simulink model "DCDC_SEPIC_TopLevelModel_Dashboard"  (R2023b)
settings: Solver=daessc  StartTime=0.0  StopTime=10  FixedStep=ts500us  MaxStep=1  RelTol=1e-3
undefined symbols (not defined in the file): NrLEDStrips, operatingMode, ts1ms, ts500us
libraries: SEPIC_utilities x6, simulink x1
settings Model: Creator=vlenzi  LastModifiedBy=vlenzi
settings SolverCC: AlgebraicLoopSolver=TrustRegion  DecoupledContinuousIntegration=on
settings DataIOCC: SaveFormat=StructureWithTime  SaveOutput=off  SaveTime=off  SignalLoggingName=logsOut
settings OptimizationCC: DefaultParameterBehavior=Inlined  UseDivisionForNetSlopeComputation=UseDivisionForReciprocalsOfIntegersOnly  ReuseModelBlockBuffer=off  EnhancedBackFolding=on  BooleansAsBitfields=on  PassReuseOutputArgsAs=Individual arguments  ExpressionDepthLimit=2147483647  StateBitsets=on  DataBitsets=on  ZeroExternalMemoryAtStartup=off  NoFixptDivByZeroProtection=on  EfficientFloat2IntCast=on  LifeSpan=1  MaxStackSize=64  SimCompilerOptimization=on  EfficientTunableParamExpr=on
settings DebuggingCC: ReadBeforeWriteMsg=DisableAll  WriteAfterWriteMsg=DisableAll  WriteAfterReadMsg=DisableAll  UnderspecifiedInitializationDetection=Classic  CheckExecutionContextPreStartOutputMsg=on  ParameterPrecisionLossMsg=none  FcnCallInpInsideContextMsg=warning  UnconnectedInputMsg=warning  UnconnectedOutputMsg=warning  UnconnectedLineMsg=warning  UniqueDataStoreMsg=error  AllowSymbolicDim=off  ModelReferenceSymbolNameMessage=none  StateNameClashWarn=warning  StrictBusMsg=ErrorOnBusTreatedAsVector  SymbolicDimsDataTypeCodeGenerationDiagnostic=none  SFUnexpectedBacktrackingDiag=warning  SFNoUnconditionalDefaultTransitionDiag=warning  SFExecutionAtInitializationDiag=none  ArithmeticOperatorsInVariantConditions=warning
settings HardwareCC: TargetHWDeviceType=Generic->32-bit Embedded Processor
settings ModelReferenceCC: EnableRefExpFcnMdlSchedulingChecks=on  CheckModelReferenceTargetMessage=none  PropagateSignalLabelsOutOfModel=off
settings SFSimCC: SimUseLocalCustomCode=off  MATLABDynamicMemAlloc=off
settings RTWCC: Description=Embedded Coder  SystemTargetFile=ert.tlc  TemplateMakefile=ert_default_tmf  GenerateReport=on  RTWVerbose=off  RTWUseLocalCustomCode=off  IncludeHyperlinkInReport=on  CodeExecutionProfiling=on  CodeProfilingSaveOptions=AllData  CodeProfilingInstrumentation=coarse  GenerateTraceInfo=on  GenerateTraceReport=on  GenerateTraceReportSl=on  GenerateTraceReportSf=on  GenerateTraceReportEml=on  GenerateCodeMetricsReport=on  DLArmComputeVersion=19.05
settings CodeAppCC: ForceParamTrailComments=on  IgnoreCustomStorageClasses=off  SimulinkDataObjDesc=on  CustomSymbolStrGlobalVar=rt$N$M  CustomSymbolStrType=$N$M  CustomSymbolStrFcn=$N$M$F  CustomSymbolStrMacro=$N$M  InsertBlockDesc=on  StateflowObjectComments=on  InternalIdentifier=Classic
settings ERTTargetCC: UtilityFuncGeneration=Shared location  MultiwordLength=2048  IncludeMdlTerminateFcn=off  CombineSignalStateStructs=on  SupportNonFinite=off  SupportComplex=off  ExtModeStaticAllocSize=2048  ERTCustomFileTemplate=example_file_process.tlc  ERTFilePackagingFormat=CompactWithDataFile  ConvertIfToSwitch=off  SuppressUnreachableDefaultCases=off
settings ConfigComp: CovMetricSettings=dw  CovSaveCumulativeToWorkspaceVar=on  CovSaveSingleToWorkspaceVar=on  CovExternalEMLEnable=off  CovSFcnEnable=off
settings SimscapeCC: SimscapeUseOperatingPoints=on  SimscapeOperatingPoint=op_tm_average

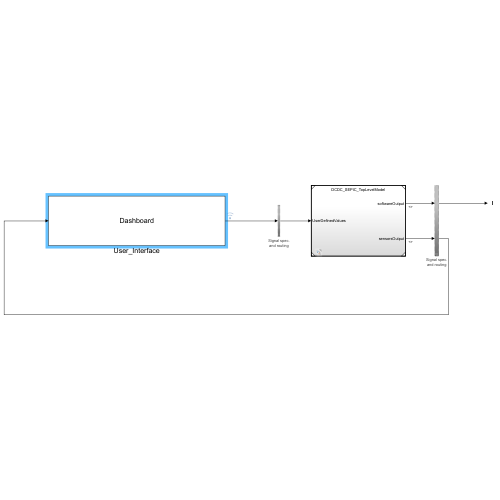
[thumbnail: Simulink's stored preview of the top-level diagram]
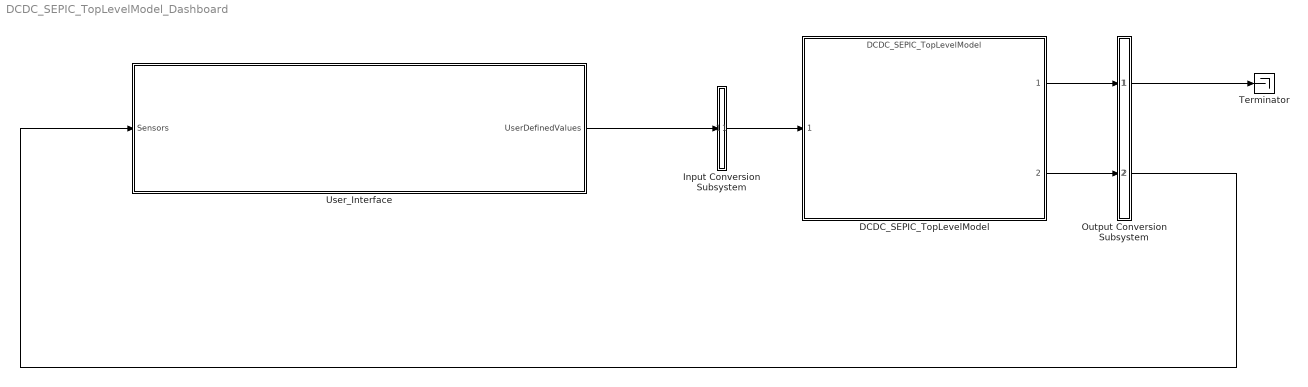
== system DCDC_SEPIC_TopLevelModel_Dashboard ==
  DCDC_SEPIC_TopLevelModel : ModelReference  ModelNameDialog=DCDC_SEPIC_TopLevelModel  SimulationMode=Normal  ModelReferenceVersion=8.30
  Input Conversion Subsystem : Subsystem  Tag=__SLT_ICS__  Description=|
      | Signal spec.
      | and routing
      settings: AttributesFormatString=%<Description>
  Output Conversion Subsystem : Subsystem  Tag=__SLT_OCS__  Description=|
      | Signal spec.
      | and routing
      settings: AttributesFormatString=%<Description>
  Terminator : Terminator
  User_Interface : Subsystem
      mask Display: disp('Dashboard')
  wires:
  Input Conversion Subsystem/1(Outport_1) -> DCDC_SEPIC_TopLevelModel/1
  DCDC_SEPIC_TopLevelModel/1 -> Output Conversion Subsystem/1(Inport_1)
  DCDC_SEPIC_TopLevelModel/2 -> Output Conversion Subsystem/2(Inport_2)
  User_Interface/1(UserDefinedValues) -> Input Conversion Subsystem/1(Inport_1)
  Output Conversion Subsystem/2(Outport_2) -> User_Interface/1(Sensors)
  Output Conversion Subsystem/1(Outport_1) -> Terminator/1

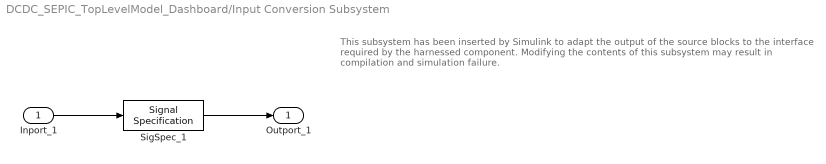
== system DCDC_SEPIC_TopLevelModel_Dashboard/Input Conversion Subsystem ==
  note: This subsystem has been inserted by Simulink to adapt the output of the source blocks to the interface required by the harnessed component.
      |  Modifying the contents of this subsystem may result in compilation and simulation failure.
  Inport_1 : Inport
  SigSpec_1 : SignalSpecification  OutDataTypeStr=Bus: UserDefinedValues  SampleTime=0.0005
  Outport_1 : Outport
  wires:
  SigSpec_1/1 -> Outport_1/1
  Inport_1/1 -> SigSpec_1/1

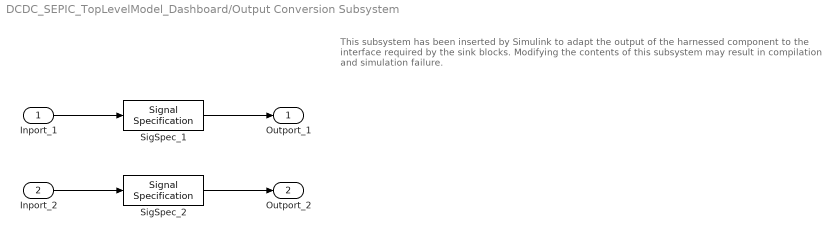
== system DCDC_SEPIC_TopLevelModel_Dashboard/Output Conversion Subsystem ==
  note: This subsystem has been inserted by Simulink to adapt the output of the harnessed component to the interface required by the sink blocks.
      |  Modifying the contents of this subsystem may result in compilation and simulation failure.
  Inport_1 : Inport
  Inport_2 : Inport  Port=2
  SigSpec_1 : SignalSpecification  OutDataTypeStr=Bus: AppSoftware  Dimensions=[1]  SampleTime=0.001
  SigSpec_2 : SignalSpecification  OutDataTypeStr=Bus: Sensors  Dimensions=[1]  SampleTime=0.0005
  Outport_1 : Outport
  Outport_2 : Outport  Port=2
  wires:
  Inport_1/1 -> SigSpec_1/1
  SigSpec_1/1 -> Outport_1/1
  Inport_2/1 -> SigSpec_2/1
  SigSpec_2/1 -> Outport_2/1

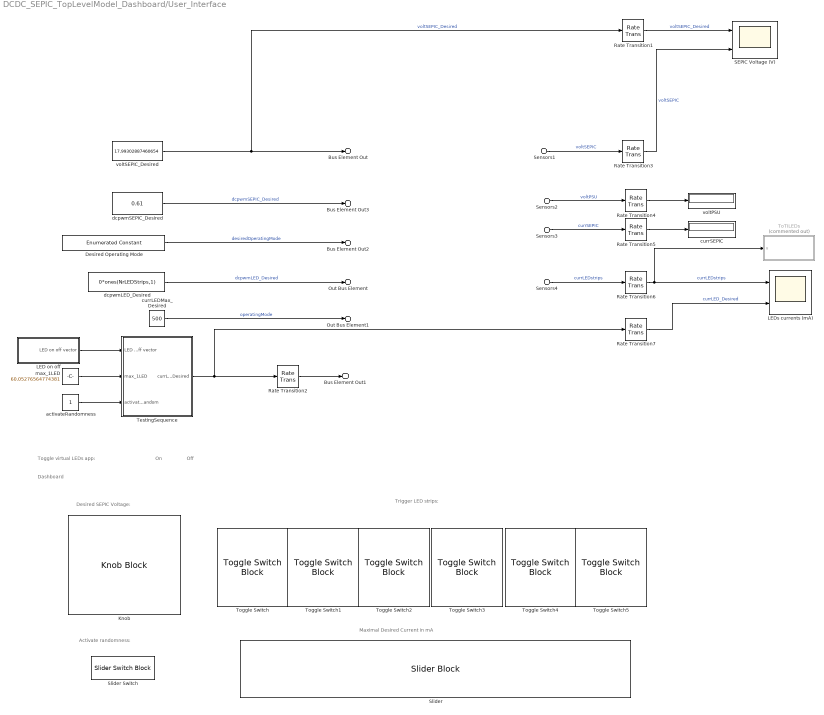
== system DCDC_SEPIC_TopLevelModel_Dashboard/User_Interface ==
  note: Maximal Desired Current in mA
  note: Dashboard
  note: Trigger LED strips:
  note: Desired SEPIC Voltage:
  note: Activate randomness:
  note: Toggle virtual LEDs app:
  note: On
  note: Off
  Sensors1 : Inport  PortName=Sensors  Element=voltSEPIC
  Sensors3 : Inport  PortName=Sensors  Element=currSEPIC
  Sensors4 : Inport  PortName=Sensors  Element=currLEDstrips
  Sensors2 : Inport  PortName=Sensors  Element=voltPSU
  Desired Operating Mode : simulink/Sources/Enumerated Constant  OutDataTypeStr=Enum: operatingMode  Value=operatingMode.AutomaticOperation  SampleTime=inf
  Knob : KnobBlock  LabelPosition=Hide  ScaleMin=9  ScaleMax=21  TickInterval=3
  LED on off : Subsystem
  LEDs currents (mA) : Scope  NumInputPorts=2
  Rate Transition{1,3..7} (6 alike) : RateTransition  Deterministic=off  OutPortSampleTime=ts10ms
  Rate Transition2 : RateTransition  Deterministic=off
  SEPIC Voltage (V) : Scope  NumInputPorts=2
  Slider : SliderBlock  LabelPosition=Hide  TickInterval=10
  Slider Switch : SliderSwitchBlock  LabelPosition=Hide
      settings: Values={{'Off', 'On'}, [0 1]}
  TestingSequence : Subsystem  Variant=on  VariantControlMode=label  VariantControl=Choice  LabelModeActiveChoice=Choice_1
  ToTILEDs : MATLAB Function  Commented=on  TreatAsAtomicUnit=on
  Toggle Switch{,1..5} (6 alike) : ToggleSwitchBlock  LabelPosition=Hide
      settings: Values={{'Off', 'On'}, [0 1]}
  activateRandomness : Constant  OutDataTypeStr=single
  currLEDMax_Desired : Constant  Value=500  OutDataTypeStr=single
  currSEPIC : Display
  dcpwmLED_Desired : Constant  Value=0*ones(NrLEDStrips,1)  OutDataTypeStr=single
  dcpwmSEPIC_Desired : Constant  Value=0.61  OutDataTypeStr=single
  max_1LED : Constant  Value=60.05276564774381  OutDataTypeStr=single
  voltPSU : Display
  voltSEPIC_Desired : Constant  Value=17.99302887460654  OutDataTypeStr=single
  Bus Element Out : Outport  PortName=UserDefinedValues  Element=voltSEPIC_Desired
  Bus Element Out1 : Outport  PortName=UserDefinedValues  Element=currLED_Desired
  Bus Element Out2 : Outport  PortName=UserDefinedValues  Element=desiredOperatingMode
  Bus Element Out3 : Outport  PortName=UserDefinedValues  Element=dcpwmSEPIC_Desired
  Out Bus Element : Outport  PortName=UserDefinedValues  Element=dcpwmLED_Desired
  Out Bus Element1 : Outport  PortName=UserDefinedValues  Element=currLEDMax_Desired
  wires:
  voltSEPIC_Desired/1 -> Bus Element Out/1, Rate Transition1/1  "voltSEPIC_Desired"
  Desired Operating Mode/1 -> Bus Element Out2/1  "desiredOperatingMode"
  Sensors1/1 -> Rate Transition3/1  "voltSEPIC"
  Sensors2/1 -> Rate Transition4/1  "voltPSU"
  Sensors3/1 -> Rate Transition5/1  "currSEPIC"
  Sensors4/1 -> Rate Transition6/1  "currLEDstrips"
  dcpwmSEPIC_Desired/1 -> Bus Element Out3/1  "dcpwmSEPIC_Desired"
  dcpwmLED_Desired/1 -> Out Bus Element/1  "dcpwmLED_Desired"
  Rate Transition6/1 -> LEDs currents (mA)/1, ToTILEDs/1(u)  "currLEDstrips"
  currLEDMax_Desired/1 -> Out Bus Element1/1  "operatingMode"
  Rate Transition3/1 -> SEPIC Voltage (V)/2  "voltSEPIC"
  Rate Transition4/1 -> voltPSU/1
  Rate Transition5/1 -> currSEPIC/1
  Rate Transition1/1 -> SEPIC Voltage (V)/1  "voltSEPIC_Desired"
  TestingSequence/1(currLED_Desired) -> Rate Transition2/1, Rate Transition7/1
  Rate Transition7/1 -> LEDs currents (mA)/2  "currLED_Desired"
  max_1LED/1 -> TestingSequence/2(max_1LED)
  LED on off/1(LED on off vector) -> TestingSequence/1(LED on off vector)
  activateRandomness/1 -> TestingSequence/3(activateRandom)
  Rate Transition2/1 -> Bus Element Out1/1

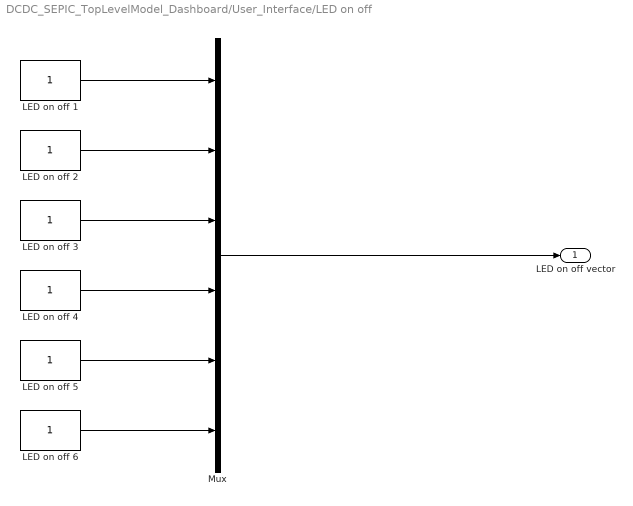
== system DCDC_SEPIC_TopLevelModel_Dashboard/User_Interface/LED on off ==
  LED on off {1..6} (6 alike) : Constant  OutDataTypeStr=single
  Mux : Mux  Inputs=6
  LED on off vector : Outport
  wires:
  Mux/1 -> LED on off vector/1
  LED on off 6/1 -> Mux/6
  LED on off 2/1 -> Mux/2
  LED on off 4/1 -> Mux/4
  LED on off 1/1 -> Mux/1
  LED on off 5/1 -> Mux/5
  LED on off 3/1 -> Mux/3

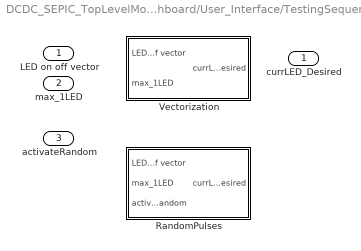
== system DCDC_SEPIC_TopLevelModel_Dashboard/User_Interface/TestingSequence ==
  LED on off vector : Inport
  max_1LED : Inport  Port=2
  activateRandom : Inport  Port=3
  RandomPulses : Subsystem  VariantControl=Choice_1
  Vectorization : Subsystem  VariantControl=Choice
  currLED_Desired : Outport

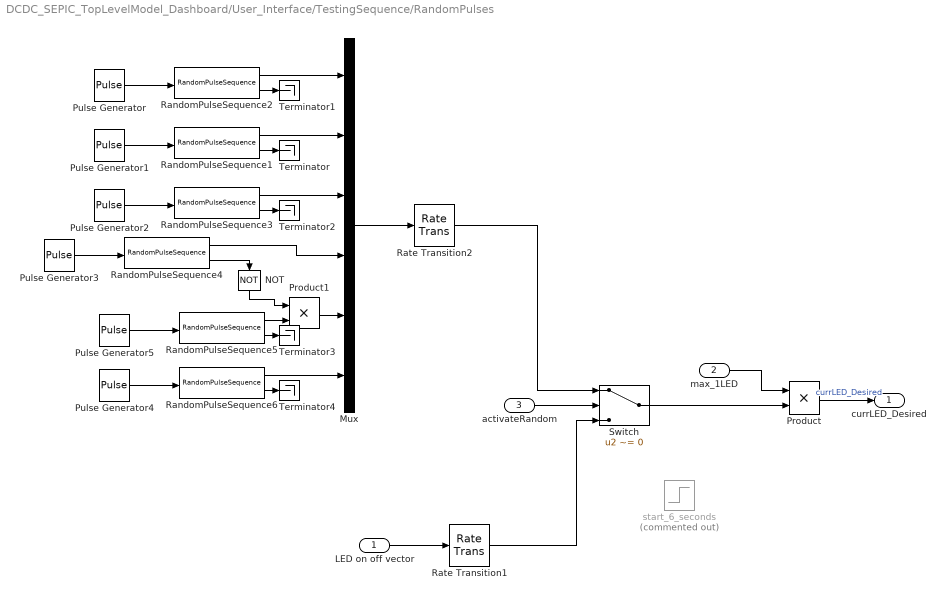
== system DCDC_SEPIC_TopLevelModel_Dashboard/User_Interface/TestingSequence/RandomPulses ==
  LED on off vector : Inport
  max_1LED : Inport  Port=2
  activateRandom : Inport  Port=3
  Mux : Mux  Inputs=6
  NOT : Logic  Operator=NOT  AllPortsSameDT=off  OutDataTypeStr=boolean
  Product : Product  OutDataTypeStr=single
  Product1 : Product
  Pulse Generator : DiscretePulseGenerator  Period=2*(1/ts500us)  PulseWidth=1*(1/ts500us)  SampleTime=ts500us
  Pulse Generator1 : DiscretePulseGenerator  Period=2*(1/ts500us)  PulseWidth=1*(1/ts500us)  PhaseDelay=1*400  SampleTime=ts500us
  Pulse Generator2 : DiscretePulseGenerator  Period=2*(1/ts500us)  PulseWidth=1*(1/ts500us)  PhaseDelay=2*400  SampleTime=ts500us
  Pulse Generator3 : DiscretePulseGenerator  Period=2*(1/ts500us)  PulseWidth=1*(1/ts500us)  PhaseDelay=3*400  SampleTime=ts500us
  Pulse Generator4 : DiscretePulseGenerator  Period=2*(1/ts500us)  PulseWidth=1*(1/ts500us)  PhaseDelay=5*400  SampleTime=ts500us
  Pulse Generator5 : DiscretePulseGenerator  Period=2*(1/ts500us)  PulseWidth=1*(1/ts500us)  PhaseDelay=4*400  SampleTime=ts500us
  RandomPulseSequence1 : SEPIC_utilities/RandomPulseSequence  seed=2  sampleTime=4
  RandomPulseSequence2 : SEPIC_utilities/RandomPulseSequence  seed=1  sampleTime=4
  RandomPulseSequence3 : SEPIC_utilities/RandomPulseSequence  seed=3  sampleTime=4
  RandomPulseSequence4 : SEPIC_utilities/RandomPulseSequence  seed=4  sampleTime=4
  RandomPulseSequence5 : SEPIC_utilities/RandomPulseSequence  seed=5  sampleTime=4
  RandomPulseSequence6 : SEPIC_utilities/RandomPulseSequence  seed=6  sampleTime=4
  Rate Transition1 : RateTransition  Deterministic=off
  Rate Transition2 : RateTransition  Deterministic=off
  Switch : Switch  Criteria=u2 ~= 0  SaturateOnIntegerOverflow=off  InputSameDT=off
  Terminator{,1..4} (5 alike) : Terminator
  start_6_seconds : Step  Commented=on  Time=6  SampleTime=ts1ms
  currLED_Desired : Outport
  wires:
  RandomPulseSequence5/2 -> Terminator3/1
  RandomPulseSequence6/2 -> Terminator4/1
  RandomPulseSequence6/1 -> Mux/6
  RandomPulseSequence2/2 -> Terminator1/1
  Pulse Generator3/1 -> RandomPulseSequence4/1
  Pulse Generator/1 -> RandomPulseSequence2/1
  RandomPulseSequence1/1 -> Mux/2
  Product1/1 -> Mux/5
  Pulse Generator2/1 -> RandomPulseSequence3/1
  RandomPulseSequence4/1 -> Mux/4
  RandomPulseSequence3/1 -> Mux/3
  RandomPulseSequence4/2 -> NOT/1
  RandomPulseSequence1/2 -> Terminator/1
  NOT/1 -> Product1/1
  Pulse Generator1/1 -> RandomPulseSequence1/1
  Pulse Generator5/1 -> RandomPulseSequence5/1
  Mux/1 -> Rate Transition2/1
  Pulse Generator4/1 -> RandomPulseSequence6/1
  RandomPulseSequence5/1 -> Product1/2
  RandomPulseSequence2/1 -> Mux/1
  RandomPulseSequence3/2 -> Terminator2/1
  Product/1 -> currLED_Desired/1  "currLED_Desired"
  max_1LED/1 -> Product/1
  activateRandom/1 -> Switch/2
  Switch/1 -> Product/2
  LED on off vector/1 -> Rate Transition1/1
  Rate Transition2/1 -> Switch/1
  Rate Transition1/1 -> Switch/3

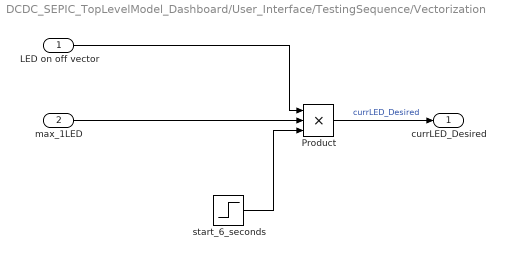
== system DCDC_SEPIC_TopLevelModel_Dashboard/User_Interface/TestingSequence/Vectorization ==
  LED on off vector : Inport
  max_1LED : Inport  Port=2
  Product : Product  Inputs=3  OutDataTypeStr=single
  start_6_seconds : Step  Time=6  SampleTime=ts1ms
  currLED_Desired : Outport
  wires:
  start_6_seconds/1 -> Product/3
  Product/1 -> currLED_Desired/1  "currLED_Desired"
  max_1LED/1 -> Product/2
  LED on off vector/1 -> Product/1

== matlab function DCDC_SEPIC_TopLevelModel_Dashboard/User_Interface/ToTILEDs ==
  data: u input
function fcn(u)
%%%%%%%%%%%%%%%%%%%%%%%%%%%%%%%%%%%%%%%%%%%%%%%%%%%%%%%%%%%%%%%%%%%%%%%%%%%%%%%%
% Function: fcn()
% Goal    : Write new values to the groups of LEDs
% IN      : - u : vector of new values for each LEDs groups
% IN/OUT  : -
% OUT     : -
%%%%%%%%%%%%%%%%%%%%%%%%%%%%%%%%%%%%%%%%%%%%%%%%%%%%%%%%%%%%%%%%%%%%%%%%%%%%%%%%
  coder.extrinsic('evalin');
  appObj = evalin('base','objLEDs');
  funObj = 'setTiLeds';
  % Write new values to each LEDs group
  for n=1:1:length(u)
    feval(funObj,appObj,u(n),n);
  end
end
